simulink library "libbestfx"  (R2018b)
settings: Solver=VariableStepAuto  StartTime=0.0  StopTime=10.0  RelTol=1e-3
undefined symbols (not defined in the file or in its folder): R, S, VariantTypeR, VariantTypeS
libraries: simulink x25, $bdroot x14
(part 1 of 2)
settings Model: Creator=Timo Fix  LastModifiedBy=tfix

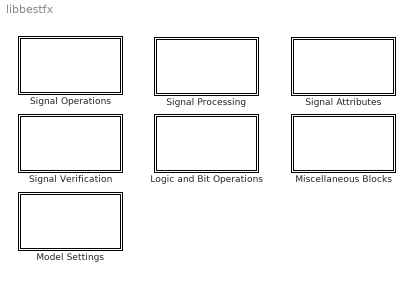
== system libbestfx ==
  Logic and Bit Operations : Subsystem
      mask Display:
      | color('white');
      | text(.1,.5,...
      |     ['\fontsize{18}me.'...
      |      '\fontsize{12}\fontname{courier}' newline ...
      |      'BitOps'],...
      |      'horizontalAlignment','left','texmode','on');
  Miscellaneous Blocks : Subsystem
      mask Display:
      | color('white');
      | text(.1,.5,...
      |     ['\fontsize{18}me.'...
      |      '\fontsize{12}\fontname{courier}' newline ...
      |      'Misc'],...
      |      'horizontalAlignment','left','texmode','on');
  Model Settings : Subsystem
      mask Display:
      | color('white');
      | text(.1,.5,...
      |     ['\fontsize{18}me.'...
      |      '\fontsize{12}\fontname{courier}' newline ...
      |      'Settings'],...
      |      'horizontalAlignment','left','texmode','on');
  Signal Attributes : Subsystem
      mask Display:
      | color('white');
      | text(.1,.5,...
      |     ['\fontsize{18}me.'...
      |      '\fontsize{12}\fontname{courier}' newline ...
      |      'SigAttr'],...
      |      'horizontalAlignment','left','texmode','on');
  Signal Operations : Subsystem
      mask Display:
      | color('white');
      | text(.1,.5,...
      |     ['\fontsize{18}me.'...
      |      '\fontsize{12}\fontname{courier}' newline ...
      |      'SigOps'],...
      |      'horizontalAlignment','left','texmode','on');
  Signal Processing : Subsystem
      mask Display:
      | color('white');
      | text(.1,.5,...
      |     ['\fontsize{18}me.'...
      |      '\fontsize{12}\fontname{courier}' newline ...
      |      'SigProc'],...
      |      'horizontalAlignment','left','texmode','on');
  Signal Verification : Subsystem
      mask Display:
      | color('white');
      | text(.1,.5,...
      |     ['\fontsize{18}me.'...
      |      '\fontsize{12}\fontname{courier}' newline ...
      |      'V&V'],...
      |      'horizontalAlignment','left','texmode','on');

== system libbestfx/Logic and Bit Operations ==
  Byte Creator : Subsystem  mask(ByteCreator me.){}
      mask help: Creates a byte composed of 8 bits.
      mask DialogControl ContainerLabel Prompt: Bit data width labels
      mask DialogControl TextLabelGroup1 Prompt: <b>Bit</b>: 1 bit<br> <b>Nibble</b>: 4 bits<br> <b>Byte</b>: 8 bits
      mask DialogControl TextLabelGroup2 Prompt: <b>Word</b>: 16 bits<br> <b>Double-Word</b>: 32 bits<br> <b>Long-Word</b>: 64 bits
  Byte Join : Subsystem  mask(ByteJoin me.){}
      mask help: Join two bytes to a word.
  Double-Word Creator : Subsystem  mask(DoubleWordCreator me.){}
      mask help: Creates a double-word composed of 32 bits.
      mask DialogControl ContainerLabel Prompt: Bit data width labels
      mask DialogControl TextLabelGroup1 Prompt: <b>Bit</b>: 1 bit<br> <b>Nibble</b>: 4 bits<br> <b>Byte</b>: 8 bits
      mask DialogControl TextLabelGroup2 Prompt: <b>Word</b>: 16 bits<br> <b>Double-Word</b>: 32 bits<br> <b>Long-Word</b>: 64 bits
  Double-Word Join : Subsystem  mask(DoubleWordJoin me.){}
      mask help: Join two double-words to a long-word.
  Nibble Creator : Subsystem  mask(NibbleCreator me.){}
      mask help: Creates a nibble composed of 4 bits.
      mask DialogControl ContainerLabel Prompt: Bit data width labels
      mask DialogControl TextLabelGroup1 Prompt: <b>Bit</b>: 1 bit<br> <b>Nibble</b>: 4 bits<br> <b>Byte</b>: 8 bits
      mask DialogControl TextLabelGroup2 Prompt: <b>Word</b>: 16 bits<br> <b>Double-Word</b>: 32 bits<br> <b>Long-Word</b>: 64 bits
  Nibble Join : Subsystem  mask(NibbleJoin me.){}
      mask help: Join two nibbles to a byte.
  Word Creator : Subsystem  mask(WordCreator me.){}
      mask help: Creates a word composed of 16 bits.
      mask DialogControl ContainerLabel Prompt: Bit data width labels
      mask DialogControl TextLabelGroup1 Prompt: <b>Bit</b>: 1 bit<br> <b>Nibble</b>: 4 bits<br> <b>Byte</b>: 8 bits
      mask DialogControl TextLabelGroup2 Prompt: <b>Word</b>: 16 bits<br> <b>Double-Word</b>: 32 bits<br> <b>Long-Word</b>: 64 bits
  Word Join : Subsystem  mask(WordJoin me.){}
      mask help: Join two words to a double-word.

== system libbestfx/Miscellaneous Blocks ==
  Continuous To Discrete : Subsystem  mask(ContinuousToDiscrete me.){Quantity=2, OutportDataType=Inherit: Inherit via back propagation, OutputPortSampleTime=-1}
      mask prompts: Quantity "Quantity Conversions:"; OutportDataType "Datatype of newly added outputs:"; OutputPortSampleTime "Output port sample time:"
      mask help: Convert continuous signals to discrete
      mask init:
      | me.sl.mask.ContinuousDiscrete();
      settings: CopyFcn=try;set(gcbh,'LinkStatus','none');end
      mask Display: plot([0 1], [0 1]);
  Discrete To Continuous : Subsystem  mask(DiscreteToContinuous me.){Quantity=2, OutportDataType=double, OutputPortSampleTime=-1}
      mask prompts: Quantity "Quantity Conversions:"; OutportDataType "Datatype of newly added outputs:"; OutputPortSampleTime "Output port sample time:"
      mask help: Convert discrete signals to continuous
      mask init:
      | me.sl.mask.ContinuousDiscrete();
      settings: CopyFcn=try;set(gcbh,'LinkStatus','none');end
      mask Display: plot([0 1], [0 1]);

== system libbestfx/Model Settings ==
  Design Block : Subsystem  InitFcn=|  mask(DesignBlock me.){blockver=V1.0}
      | if me.sl.style.DEBUG
      |     fprintf('%s::DesignBlock: apply style\n',me.sl.cfg.meSimulinkLibraryName());
      | end
      | me.sl.style.apply();
      mask prompts: blockver "Design Guideline Version"
      settings: OpenFcn=|
      | if me.sl.style.DEBUG
      |     fprintf('tsflib::DesignBlock: apply style\n');
      | end
      | me.sl.style.apply();
      mask TypeOptions blockver: V1.0
      mask Display:
      | color('black');
      | text(.1,.5,...
      |     ['\fontsize{18}me.'...
      |      '\fontsize{12}\fontname{courier}' newline ...
      |      'Apply Style'],...
      |      'horizontalAlignment','left','texmode','on');

== system libbestfx/Signal Attributes ==
  Data Pack : Subsystem  mask(DataPack .me){BlockSubtypeVariant=Unsigned, Length=8, Scale=1, Offset=0, ScaleDataType=Inherit: Inherit from 'Constant value', OffsetDataType=Inherit: Inherit from 'Constant value', OutputDataType=Inherit: Inherit via back propagation}
      mask prompts: BlockSubtypeVariant "Bit Specifier:"; Length "Length (Quantity Of Bits):"; Scale "Scale (Resolution Per Bit):"; Offset "Offset (Scaled):"; ScaleDataType "Scale:"; OffsetDataType "Offset:"
      mask help: Packs a physical or numerical signal (u) into a compressed equivalent in raw format (y, quantized signal with scaling and offset), using the specified parameters.
      mask init:
      | me.sl.mask.datapack();
      settings: AttributesFormatString=8 Unsigned Bits
      mask TypeOptions BlockSubtypeVariant: Unsigned | Signed | Floating-Point
      mask DialogControl TabParam Prompt: Main
      mask DialogControl Length Tooltip: Expect positive regular numeric value.
      mask DialogControl Scale Tooltip: Expect positive regular numeric value.
      mask DialogControl Offset Tooltip: Expect non-negative regular numeric value.
      mask DialogControl TabType Prompt: Parameter Attributes
      mask DialogControl TextType Prompt: The 'OutputDataType' specifies the desired datatype for this block. Please make sure that the data types of all parameters are identical.
      mask DialogControl TextTypeNote Prompt: <i style="color:blue">Note: In the case of back propagation, it should be considered that the numerical value in the runtime data type may not be represented correctly.</i>
      mask DialogControl TabMode Prompt: Info
      mask DialogControl TextModeCounter Prompt: <b>Counter:</b> Counts up immediately as soon as the counting unit has been activated, e.g. an 'Upper Limit' of ten is reached after nine counting steps.
      mask DialogControl TextModeTimer Prompt: <b>Timer:</b> Counts the elapsed counting steps when the counting unit is activated, e.g. an 'Upper Limit' of ten is reached after ten counting steps.
      mask DialogControl TextModeOptionFreeRunning Prompt: The option <b>Free-Running</b>: The counting unit is automatically reset after the status of the counting unit is active. The status is kept active for one cycle followed by a reset cycle.
      mask DialogControl TextModeOptionBidirectional Prompt: The option <b>Bidirectional</b>: After the status of the counting unit is active, it is held. The state is not reset to false until the count of the counting unit has dropped to zero again.
      mask DialogControl TextModeNote Prompt: <br><i style="color:blue;">Note: The internal counter and initial value cannot become negative, because they are saturated to zero.</i>
      mask Display: disp('pack');
  Data Unpack : Subsystem  mask(DataUnpack .me){BlockSubtypeVariant=Unsigned, Length=8, Scale=1, Offset=0, ScaleDataType=Inherit: Inherit from 'Constant value', OffsetDataType=Inherit: Inherit from 'Constant value', OutputDataType=Inherit: Inherit via back propagation}
      mask prompts: BlockSubtypeVariant "Bit Specifier:"; Length "Length (Quantity Of Bits):"; Scale "Scale (Resolution Per Bit):"; Offset "Offset (Scaled):"; ScaleDataType "Scale:"; OffsetDataType "Offset:"
      mask help: unpack a signal in raw format (u, quantized signal with scaling and offset) to its physical or numerical original equivalent (y), using the specified parameters.
      mask init:
      | me.sl.mask.datapack();
      settings: AttributesFormatString=8 Unsigned Bits
      mask TypeOptions BlockSubtypeVariant: Unsigned | Signed | Floating-Point
      mask DialogControl TabParam Prompt: Main
      mask DialogControl Length Tooltip: Expect positive regular numeric value.
      mask DialogControl Scale Tooltip: Expect positive regular numeric value.
      mask DialogControl Offset Tooltip: Expect non-negative regular numeric value.
      mask DialogControl TabType Prompt: Parameter Attributes
      mask DialogControl TextType Prompt: The 'Scale' specifies the desired datatype for this block. Please make sure that the data types of all parameters are identical.
      mask DialogControl TextTypeNote Prompt: <i style="color:blue">Note: In the case of back propagation, it should be considered that the numerical value in the runtime data type may not be represented correctly.</i>
      mask DialogControl TabMode Prompt: Info
      mask DialogControl TextModeCounter Prompt: <b>Counter:</b> Counts up immediately as soon as the counting unit has been activated, e.g. an 'Upper Limit' of ten is reached after nine counting steps.
      mask DialogControl TextModeTimer Prompt: <b>Timer:</b> Counts the elapsed counting steps when the counting unit is activated, e.g. an 'Upper Limit' of ten is reached after ten counting steps.
      mask DialogControl TextModeOptionFreeRunning Prompt: The option <b>Free-Running</b>: The counting unit is automatically reset after the status of the counting unit is active. The status is kept active for one cycle followed by a reset cycle.
      mask DialogControl TextModeOptionBidirectional Prompt: The option <b>Bidirectional</b>: After the status of the counting unit is active, it is held. The state is not reset to false until the count of the counting unit has dropped to zero again.
      mask DialogControl TextModeNote Prompt: <br><i style="color:blue;">Note: The internal counter and initial value cannot become negative, because they are saturated to zero.</i>
      mask Display: disp('unpack');
  Overwrite : Subsystem  mask(Overwrite .me){val=0.0}
      mask prompts: val "Overwrite value:"
      mask help: Overwrite the incoming signal value. Other signal properties like data type and dimension remain unchanged.
      mask Display: fprintf('y = %g',val)
  Rename : Subsystem  mask(Rename .me){}
      mask help: Renaming of the incoming signal. Other signal properties such as data type and dimension remain unchanged.
      mask Display: disp('rename');

== system libbestfx/Signal Operations ==
  Counter Timer Unit : Subsystem  mask(CounterTimerUnit .me){BlockSubtypeVariant=Counter, UpperLimitSourcePort=off, EnableSourcePort=on, IncrementSourcePort=off, DecrementSourcePort=off, InitialConditionSourcePort=off, ResetSourcePort=off, CounterTimerStateSinkPort=on, CounterTimerValueSinkPort=off, UpperLimit=10, Increment=1, Decrement=0, InitialCondition=0, UpperLimitDataType=Inherit: Inherit from 'Constant value', IncrementDataType=Inherit: Inherit from 'Constant value', DecrementDataType=Inherit: Inherit from 'Constant value', InitialConditionDataType=Inherit: Inherit from 'Constant value'}
      mask prompts: BlockSubtypeVariant "Mode:"; UpperLimitSourcePort "Show port 'Upper Limit'"; EnableSourcePort "Show port 'Enable'"; IncrementSourcePort "Show port 'Increment'"; DecrementSourcePort "Show port 'Decrement'"; InitialConditionSourcePort "Show port 'Initial Condition'"; ResetSourcePort "Show port 'Reset'"; CounterTimerStateSinkPort "Show port 'State'"; CounterTimerValueSinkPort "Show port 'Value'"; UpperLimit "Upper Limit:"; Increment "Counter Increment:"; Decrement "Counter Decrement:"; InitialCondition "Initial Condition: Limited to the value range from zero to the 'Upper Limit'."; UpperLimitDataType "Upper Limit:"; IncrementDataType "Increment:"; DecrementDataType "Decrement:"; InitialConditionDataType "Initial Condition:"
      mask help: Counter unit which counts in different ways. Two counting modes are available (counter/timer), each optionally with the option bidirectional or free-running.
      mask init:
      | me.sl.mask.countertimerunit();
      settings: AttributesFormatString=|
      | %<BlockSubtypeVariant>
      | Upper Limit: 10
      mask TypeOptions BlockSubtypeVariant: Counter | Timer | Bidirectional Counter | Bidirectional Timer | Free-Running Counter | Free-Running Timer
      mask DialogControl TabParam Prompt: Main
      mask DialogControl ContainerSources Prompt: Show Inports
      mask DialogControl ContainerSinks Prompt: Show Outports
      mask DialogControl UpperLimit Tooltip: Expect positive regular numeric value.
      mask DialogControl Increment Tooltip: Expect positive regular numeric value.
      mask DialogControl Decrement Tooltip: Expect non-negative regular numeric value.
      mask DialogControl InitialCondition Tooltip: Expect regular numeric value.
      mask DialogControl TabType Prompt: Parameter Attributes
      mask DialogControl TextType Prompt: The 'Upper Limit' specifies the desired datatype for the counting unit. Please make sure that the data types of all parameters are identical.
      mask DialogControl TextTypeNote Prompt: <i style="color:blue">Note: In the case of back propagation, it should be considered that the numerical value in the runtime data type may not be represented correctly.</i>
      mask DialogControl TabMode Prompt: Info
      mask DialogControl TextModeCounter Prompt: <b>Counter:</b> Counts up immediately as soon as the counting unit has been activated, e.g. an 'Upper Limit' of ten is reached after nine counting steps.
      mask DialogControl TextModeTimer Prompt: <b>Timer:</b> Counts the elapsed counting steps when the counting unit is activated, e.g. an 'Upper Limit' of ten is reached after ten counting steps.
      mask DialogControl TextModeOptionFreeRunning Prompt: The option <b>Free-Running</b>: The counting unit is automatically reset after the status of the counting unit is active. The status is kept active for one cycle followed by a reset cycle.
      mask DialogControl TextModeOptionBidirectional Prompt: The option <b>Bidirectional</b>: After the status of the counting unit is active, it is held. The state is not reset to false until the count of the counting unit has dropped to zero again.
      mask DialogControl TextModeNote Prompt: <br><i style="color:blue;">Note: The internal counter and initial value cannot become negative, because they are saturated to zero.</i>
  Debounce Unit : Subsystem  mask(CounterTimerUnit .me){BlockSubtypeVariant=Holding Element, SamplesSourcePort=off, Samples=10, SampleTime=-1, SamplesConversion=on, SamplesDataType=Inherit: Inherit from 'Constant value'}
      mask prompts: BlockSubtypeVariant "Mode:"; SamplesSourcePort "Show port 'Debounce Samples'"; Samples "Debounce Samples:"; SampleTime "Sample Time:"; SamplesConversion "Convert 'Debounce Samples' to time interval in seconds"; SamplesDataType "Debounce Samples:"
      mask help: Debouncing unit that suppresses fast changes of the input signal (u) in various ways. Three modes are available (holding element, switch-on delay and switch-off delay).
      mask init:
      | me.sl.mask.debounceunit();
      settings: AttributesFormatString=|
      | %<BlockSubtypeVariant>
      | 10x samples
      mask TypeOptions BlockSubtypeVariant: Holding Element | Switch-On Delay | Switch-Off Delay
      mask DialogControl TabParam Prompt: Main
      mask DialogControl ContainerSources Prompt: Show Inports
      mask DialogControl Samples Tooltip: Expect positive regular numeric value.
      mask DialogControl ContainerPreview Prompt: Block Parameter Preview
      mask DialogControl TextPreviewNote Prompt: <i style="color:blue">Note: A conversion is only possible if the 'Sample Time' is explicitly specified, which means it is not '-1'.</i>
      mask DialogControl TabType Prompt: Parameter Attributes
      mask DialogControl TabMode Prompt: Info
      mask DialogControl TextModeHoldingElement Prompt: <b>Holding Element:</b> Holds the active level for a presettable 'Debounce Samples' minimum time. After this minimum time has elapsed, the input level is passed through.
      mask DialogControl TextModeSwitchOffDelay Prompt: <b>Switch-Off Delay:</b> Holds the active level for a presettable 'Debounce Samples' hold time after the input signal is reset. The duration of this hold time restarts with each falling edge.
      mask DialogControl TextModeSwitchOnDelay Prompt: <b>Switch-On Delay:</b> Suppresses the active level of the input signal until the predefinable 'Debounce Samples' hold time has elapsed.
  Flip-Flop : Subsystem  mask(FlipFlop .me){BlockSubtypeVariant=Bistable S-R, StateSourcePort=on, NegatedStateSourcePort=off, InitialCondition=false}
      mask prompts: BlockSubtypeVariant "Mode:"; StateSourcePort "Show port 'State'"; NegatedStateSourcePort "Show port 'Negated State'"; InitialCondition "Initial Condition:"
      mask help: Bistable flip-flop without restricted combination (forbidden state). Set or reset condition is dominant as soon as both inputs are set. Two flip-flop modes are available.
      mask init:
      | me.sl.mask.flipflop();
      settings: AttributesFormatString=%<BlockSubtypeVariant>
      mask TypeOptions BlockSubtypeVariant: Bistable S-R | Bistable R-S
      mask DialogControl TabParam Prompt: Main
      mask DialogControl ContainerSinks Prompt: Show Outports
      mask DialogControl TabMode Prompt: Info
      mask DialogControl TextModeSR Prompt: <b>Bistable S-R:</b> Characterized by a dominant set condition.
      mask DialogControl TextModeRS Prompt: <b>Bistable R-S:</b> Characterized by a dominant reset condition.
      mask Display:
      | color('green');
      | port_label('input', 1, '_');
  Interactive Switch : Subsystem  mask(InteractiveSwitch .me){ctrl=off}
      mask prompts: ctrl "BUTTON"
      mask init:
      | me.sl.mask.switchinteractive();
      settings: OpenFcn=me.sl.mask.switchinteractive('clbk','openfnc')
      mask Display: disp('OFF')
  Pulse Divider : Subsystem  mask(PulseDivider me.){DivisorSourcePort=off, Divisor=2, DivisorDataType=uint8}
      mask prompts: DivisorSourcePort "Show port "Divisor""; DivisorDataType "Divisor:"
      mask help: The sequence of input pulses (u) is reduced by the divisor (k), resulting in slower output pulses (y).
      mask init:
      | me.sl.mask.pulsedivider();
      mask DialogControl TabParam Prompt: Main
      mask DialogControl ContainerSource Prompt: Show Inports
      mask DialogControl TabTypes Prompt: Parameter Attributes
  Pulse Selector : Subsystem  mask(PulseSelector me.){MaximumSourcePort=off, SubsetSourcePort=off, Maximum=5, Subset=3, MaximumDataType=uint8, SubsetDataType=uint8}
      mask prompts: MaximumSourcePort "Show port "Maximum Of Pulses""; SubsetSourcePort "Show port "Subset Of Pulses""; Maximum "Total Amount:"; Subset "Subset Amount: Limited to the value range from zero to the 'Total Amount'"; MaximumDataType "Maximum Of Pulses:"; SubsetDataType "Subset Of Pulses:"
      mask help: Starting from an ever-repeating sequence of input pulses (u), the length of the sequence is described by the maximum of pulses (nmax). Only a subset of pulses (n) are passed through. Intervening pulses are suppressed until the sequence starts from the beginning.
      mask init:
      | me.sl.mask.pulseselector();
      settings: AttributesFormatString=3 out of 5
      mask DialogControl TabParam Prompt: Main
      mask DialogControl ContainerSource Prompt: Show Inports
      mask DialogControl TabTypes Prompt: Parameter Attributes
  Switch To Zero : Subsystem  mask(SwitchToZero me.){}
      mask help: Sets the output signal (y) to zero if the input signal (TF) is set. Otherwise the input signal (u) is passed through.
      mask Display: fprintf('Zero when\nTF > 0');

== system libbestfx/Signal Processing ==
  Discrete Filter : Subsystem  mask(DiscreteFilter .me){BlockSubtypeVariant=Lowpass, FilterCoefficientSourcePort=off, InitialConditionSourcePort=off, ResetSourcePort=off, FilterCoefficient=0.97, InitialCondition=0, FilterCoefficientDataType=Inherit: Inherit from 'Constant value', InitialConditionDataType=Inherit: Inherit from 'Constant value'}
      mask prompts: BlockSubtypeVariant "Mode:"; FilterCoefficientSourcePort "Show port 'Filter Coefficient'"; InitialConditionSourcePort "Show port 'Initial Condition'"; ResetSourcePort "Show port 'Reset'"; FilterCoefficient "Filter Coefficent [0..1]:"; InitialCondition "Initial Condition:"; FilterCoefficientDataType "Filter Coefficent:"; InitialConditionDataType "Initial Condition:"
      mask help: Digital discrete signal filter. Two modes are available (lowpass/highpass).
      mask init:
      | me.sl.mask.discretefilter();
      settings: AttributesFormatString=|
      | %<BlockSubtypeVariant>
      | Filter Coefficient: 0.97
      mask TypeOptions BlockSubtypeVariant: Lowpass | Highpass
      mask DialogControl TabParam Prompt: Main
      mask DialogControl ContainerShowPorts Prompt: Show Inports
      mask DialogControl TabType Prompt: Parameter Attributes
      mask DialogControl TabMode Prompt: Info
      mask DialogControl ContainerMode Prompt: Filter Transfer Functions
      mask DialogControl TextModeLowpass Prompt: Discrete Lowpass:
      mask DialogControl TextModeHighpass Prompt: Discrete Highpass:
      mask DialogControl TextModeLowpassTransferFunction Prompt: <table><td><code><br>LP(z)=<br></code></td><td><code>1-T<br>----<br>z -T</code></td></table>
      mask DialogControl TextModeHighpassTransferFunction Prompt: <table><td><code><br>HP(z)=<br></code></td><td><code>z -1<br>----<br>z -T</code></td></table>
      mask Display: disp('LP(z)');

== system libbestfx/Signal Verification ==
  Validate : Subsystem  mask{BlockSubtypeVariant=Value Inside, LowerLimitSourcePort=off, UpperLimitSourcePort=off, LowerLimit=0, UpperLimit=1, LowerLimitDataType=Inherit: Inherit from 'Constant value', UpperLimitDataType=Inherit: Inherit from 'Constant value'}
      mask prompts: BlockSubtypeVariant "Mode:"; LowerLimitSourcePort "Show port 'Lower Limit'"; UpperLimitSourcePort "Show port 'Upper Limit'"; LowerLimit "Lower Limit:"; UpperLimit "Upper Limit:"; LowerLimitDataType "Lower Limit:"; UpperLimitDataType "Upper Limit:"
      mask init:
      | me.sl.mask.validate();
      settings: AttributesFormatString=|
      | %<BlockSubtypeVariant>
      | Interval [0 .. 1]
      mask TypeOptions BlockSubtypeVariant: Value Inside | Value Below | Value Above | Stuck | Stuck Inside | Stuck Below | Stuck Above
      mask DialogControl TabParam Prompt: Main
      mask DialogControl ContainerSources Prompt: Show Inports
      mask DialogControl ContainerSinks Prompt: Show Outports
      mask DialogControl TabType Prompt: Parameter Attributes

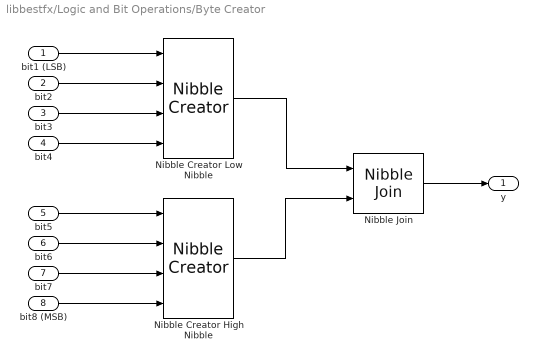
== system libbestfx/Logic and Bit Operations/Byte Creator ==
  bit1 (LSB) : Inport
  bit2 : Inport  Port=2
  bit3 : Inport  Port=3
  bit4 : Inport  Port=4
  bit5 : Inport  Port=5
  bit6 : Inport  Port=6
  bit7 : Inport  Port=7
  bit8 (MSB) : Inport  Port=8
  Nibble Creator High Nibble : $bdroot/Logic and Bit Operations/Nibble Creator
  Nibble Creator Low Nibble : $bdroot/Logic and Bit Operations/Nibble Creator
  Nibble Join : $bdroot/Logic and Bit Operations/Nibble Join
  y : Outport
  wires:
  Nibble Creator High Nibble/1 -> Nibble Join/2
  Nibble Creator Low Nibble/1 -> Nibble Join/1
  bit8 (MSB)/1 -> Nibble Creator High Nibble/4
  bit7/1 -> Nibble Creator High Nibble/3
  bit6/1 -> Nibble Creator High Nibble/2
  bit5/1 -> Nibble Creator High Nibble/1
  bit4/1 -> Nibble Creator Low Nibble/4
  bit3/1 -> Nibble Creator Low Nibble/3
  Nibble Join/1 -> y/1
  bit2/1 -> Nibble Creator Low Nibble/2
  bit1 (LSB)/1 -> Nibble Creator Low Nibble/1

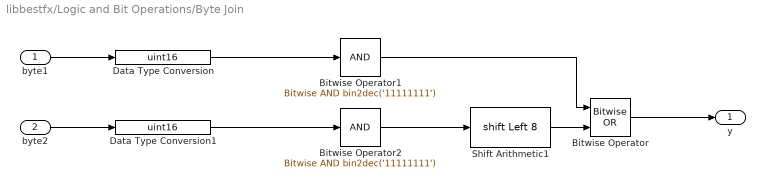
== system libbestfx/Logic and Bit Operations/Byte Join ==
  "byte1 " : Inport
  byte2 : Inport  Port=2
  Bitwise Operator : simulink/Logic and Bit Operations/Bitwise Operator  logicop=OR  UseBitMask=off  NumInputPorts=2  BitMask=bin2dec('11011001')  BitMaskRealWorld=Stored Integer
  Bitwise Operator1 : simulink/Logic and Bit Operations/Bitwise Operator  logicop=AND  UseBitMask=on  BitMask=bin2dec('11111111')  BitMaskRealWorld=Stored Integer
  Bitwise Operator2 : simulink/Logic and Bit Operations/Bitwise Operator  logicop=AND  UseBitMask=on  BitMask=bin2dec('11111111')  BitMaskRealWorld=Stored Integer
  Data Type Conversion : DataTypeConversion  OutDataTypeStr=uint16
  Data Type Conversion1 : DataTypeConversion  OutDataTypeStr=uint16
  Shift Arithmetic1 : ArithShift  BitShiftNumber=8  BitShiftDirection=Left
  y : Outport
  wires:
  byte2/1 -> Data Type Conversion1/1
  Bitwise Operator2/1 -> Shift Arithmetic1/1
  Shift Arithmetic1/1 -> Bitwise Operator/2
  Bitwise Operator1/1 -> Bitwise Operator/1
  Bitwise Operator/1 -> y/1
  Data Type Conversion/1 -> Bitwise Operator1/1
  "byte1 "/1 -> Data Type Conversion/1
  Data Type Conversion1/1 -> Bitwise Operator2/1

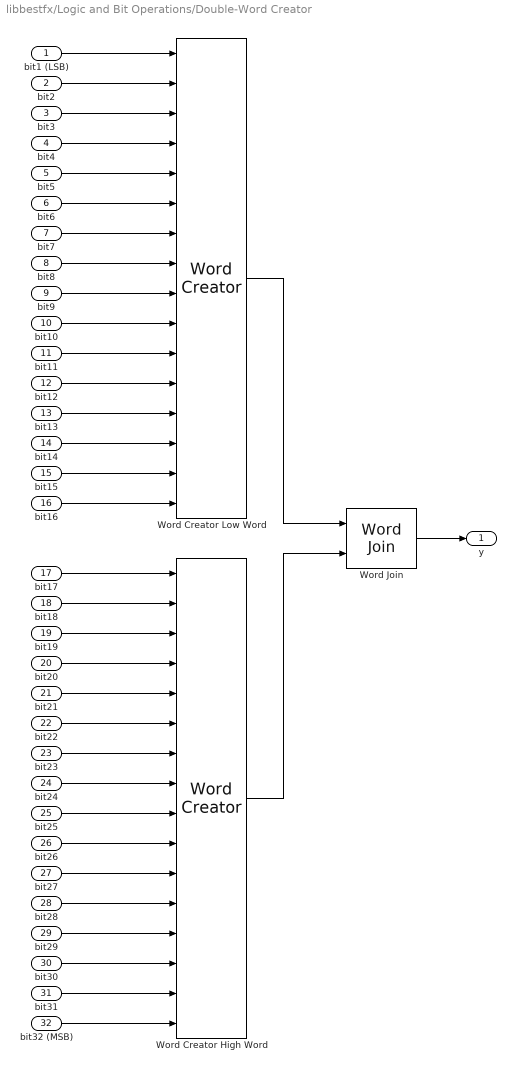
== system libbestfx/Logic and Bit Operations/Double-Word Creator ==
  bit1 (LSB) : Inport
  bit2 : Inport  Port=2
  bit3 : Inport  Port=3
  bit4 : Inport  Port=4
  bit5 : Inport  Port=5
  bit6 : Inport  Port=6
  bit7 : Inport  Port=7
  bit8 : Inport  Port=8
  bit9 : Inport  Port=9
  bit10 : Inport  Port=10
  bit11 : Inport  Port=11
  bit12 : Inport  Port=12
  bit13 : Inport  Port=13
  bit14 : Inport  Port=14
  bit15 : Inport  Port=15
  bit16 : Inport  Port=16
  bit17 : Inport  Port=17
  bit18 : Inport  Port=18
  bit19 : Inport  Port=19
  bit20 : Inport  Port=20
  bit21 : Inport  Port=21
  bit22 : Inport  Port=22
  bit23 : Inport  Port=23
  bit24 : Inport  Port=24
  bit25 : Inport  Port=25
  bit26 : Inport  Port=26
  bit27 : Inport  Port=27
  bit28 : Inport  Port=28
  bit29 : Inport  Port=29
  bit30 : Inport  Port=30
  bit31 : Inport  Port=31
  bit32 (MSB) : Inport  Port=32
  Word Creator High Word : $bdroot/Logic and Bit Operations/Word Creator
  Word Creator Low Word : $bdroot/Logic and Bit Operations/Word Creator
  Word Join : $bdroot/Logic and Bit Operations/Word Join
  y : Outport
  wires:
  bit1 (LSB)/1 -> Word Creator Low Word/1
  Word Creator High Word/1 -> Word Join/2
  Word Creator Low Word/1 -> Word Join/1
  Word Join/1 -> y/1
  bit2/1 -> Word Creator Low Word/2
  bit3/1 -> Word Creator Low Word/3
  bit4/1 -> Word Creator Low Word/4
  bit5/1 -> Word Creator Low Word/5
  bit6/1 -> Word Creator Low Word/6
  bit7/1 -> Word Creator Low Word/7
  bit8/1 -> Word Creator Low Word/8
  bit9/1 -> Word Creator Low Word/9
  bit10/1 -> Word Creator Low Word/10
  bit11/1 -> Word Creator Low Word/11
  bit12/1 -> Word Creator Low Word/12
  bit13/1 -> Word Creator Low Word/13
  bit14/1 -> Word Creator Low Word/14
  bit15/1 -> Word Creator Low Word/15
  bit16/1 -> Word Creator Low Word/16
  bit17/1 -> Word Creator High Word/1
  bit18/1 -> Word Creator High Word/2
  bit19/1 -> Word Creator High Word/3
  bit20/1 -> Word Creator High Word/4
  bit21/1 -> Word Creator High Word/5
  bit22/1 -> Word Creator High Word/6
  bit23/1 -> Word Creator High Word/7
  bit24/1 -> Word Creator High Word/8
  bit25/1 -> Word Creator High Word/9
  bit26/1 -> Word Creator High Word/10
  bit27/1 -> Word Creator High Word/11
  bit28/1 -> Word Creator High Word/12
  bit29/1 -> Word Creator High Word/13
  bit30/1 -> Word Creator High Word/14
  bit31/1 -> Word Creator High Word/15
  bit32 (MSB)/1 -> Word Creator High Word/16

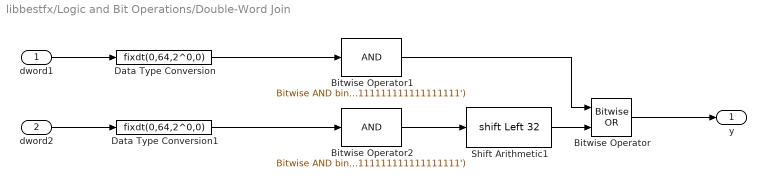
== system libbestfx/Logic and Bit Operations/Double-Word Join ==
  "dword1 " : Inport
  dword2 : Inport  Port=2
  Bitwise Operator : simulink/Logic and Bit Operations/Bitwise Operator  logicop=OR  UseBitMask=off  NumInputPorts=2  BitMask=bin2dec('11011001')  BitMaskRealWorld=Stored Integer
  Bitwise Operator1 : simulink/Logic and Bit Operations/Bitwise Operator  logicop=AND  UseBitMask=on  BitMask=bin2dec('11111111111111111111111111111111')  BitMaskRealWorld=Stored Integer
  Bitwise Operator2 : simulink/Logic and Bit Operations/Bitwise Operator  logicop=AND  UseBitMask=on  BitMask=bin2dec('11111111111111111111111111111111')  BitMaskRealWorld=Stored Integer
  Data Type Conversion : DataTypeConversion  OutDataTypeStr=fixdt(0,64,2^0,0)
  Data Type Conversion1 : DataTypeConversion  OutDataTypeStr=fixdt(0,64,2^0,0)
  Shift Arithmetic1 : ArithShift  BitShiftNumber=32  BitShiftDirection=Left
  y : Outport
  wires:
  Data Type Conversion1/1 -> Bitwise Operator2/1
  "dword1 "/1 -> Data Type Conversion/1
  Data Type Conversion/1 -> Bitwise Operator1/1
  Bitwise Operator/1 -> y/1
  Bitwise Operator1/1 -> Bitwise Operator/1
  Shift Arithmetic1/1 -> Bitwise Operator/2
  Bitwise Operator2/1 -> Shift Arithmetic1/1
  dword2/1 -> Data Type Conversion1/1

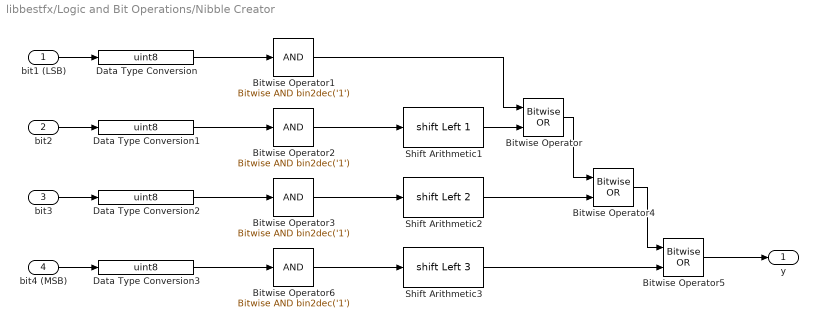
== system libbestfx/Logic and Bit Operations/Nibble Creator ==
  bit1 (LSB) : Inport
  bit2 : Inport  Port=2
  bit3 : Inport  Port=3
  bit4 (MSB) : Inport  Port=4
  Bitwise Operator : simulink/Logic and Bit Operations/Bitwise Operator  logicop=OR  UseBitMask=off  NumInputPorts=2  BitMask=bin2dec('11011001')  BitMaskRealWorld=Stored Integer
  Bitwise Operator{1..3,6} (4 alike) : simulink/Logic and Bit Operations/Bitwise Operator  logicop=AND  UseBitMask=on  BitMask=bin2dec('1')  BitMaskRealWorld=Stored Integer
  Bitwise Operator4 : simulink/Logic and Bit Operations/Bitwise Operator  logicop=OR  UseBitMask=off  NumInputPorts=2  BitMask=bin2dec('11011001')  BitMaskRealWorld=Stored Integer
  Bitwise Operator5 : simulink/Logic and Bit Operations/Bitwise Operator  logicop=OR  UseBitMask=off  NumInputPorts=2  BitMask=bin2dec('11011001')  BitMaskRealWorld=Stored Integer
  Data Type Conversion{,1..3} (4 alike) : DataTypeConversion  OutDataTypeStr=uint8
  Shift Arithmetic1 : ArithShift  BitShiftNumber=1  BitShiftDirection=Left
  Shift Arithmetic2 : ArithShift  BitShiftNumber=2  BitShiftDirection=Left
  Shift Arithmetic3 : ArithShift  BitShiftNumber=3  BitShiftDirection=Left
  y : Outport
  wires:
  bit1 (LSB)/1 -> Data Type Conversion/1
  bit2/1 -> Data Type Conversion1/1
  Bitwise Operator2/1 -> Shift Arithmetic1/1
  Bitwise Operator/1 -> Bitwise Operator4/1
  Shift Arithmetic1/1 -> Bitwise Operator/2
  Bitwise Operator1/1 -> Bitwise Operator/1
  Bitwise Operator3/1 -> Shift Arithmetic2/1
  bit3/1 -> Data Type Conversion2/1
  Shift Arithmetic2/1 -> Bitwise Operator4/2
  Shift Arithmetic3/1 -> Bitwise Operator5/2
  bit4 (MSB)/1 -> Data Type Conversion3/1
  Bitwise Operator6/1 -> Shift Arithmetic3/1
  Bitwise Operator4/1 -> Bitwise Operator5/1
  Bitwise Operator5/1 -> y/1
  Data Type Conversion/1 -> Bitwise Operator1/1
  Data Type Conversion1/1 -> Bitwise Operator2/1
  Data Type Conversion2/1 -> Bitwise Operator3/1
  Data Type Conversion3/1 -> Bitwise Operator6/1

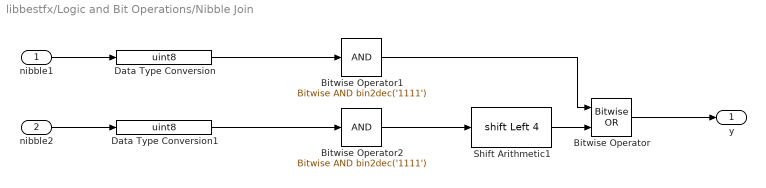
== system libbestfx/Logic and Bit Operations/Nibble Join ==
  "nibble1 " : Inport
  nibble2 : Inport  Port=2
  Bitwise Operator : simulink/Logic and Bit Operations/Bitwise Operator  logicop=OR  UseBitMask=off  NumInputPorts=2  BitMask=bin2dec('11011001')  BitMaskRealWorld=Stored Integer
  Bitwise Operator1 : simulink/Logic and Bit Operations/Bitwise Operator  logicop=AND  UseBitMask=on  BitMask=bin2dec('1111')  BitMaskRealWorld=Stored Integer
  Bitwise Operator2 : simulink/Logic and Bit Operations/Bitwise Operator  logicop=AND  UseBitMask=on  BitMask=bin2dec('1111')  BitMaskRealWorld=Stored Integer
  Data Type Conversion : DataTypeConversion  OutDataTypeStr=uint8
  Data Type Conversion1 : DataTypeConversion  OutDataTypeStr=uint8
  Shift Arithmetic1 : ArithShift  BitShiftNumber=4  BitShiftDirection=Left
  y : Outport
  wires:
  nibble2/1 -> Data Type Conversion1/1
  Bitwise Operator2/1 -> Shift Arithmetic1/1
  Shift Arithmetic1/1 -> Bitwise Operator/2
  Bitwise Operator1/1 -> Bitwise Operator/1
  Bitwise Operator/1 -> y/1
  Data Type Conversion/1 -> Bitwise Operator1/1
  "nibble1 "/1 -> Data Type Conversion/1
  Data Type Conversion1/1 -> Bitwise Operator2/1

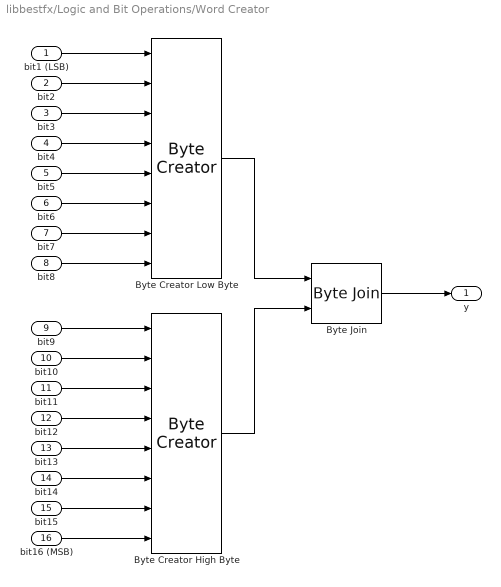
== system libbestfx/Logic and Bit Operations/Word Creator ==
  bit1 (LSB) : Inport
  bit2 : Inport  Port=2
  bit3 : Inport  Port=3
  bit4 : Inport  Port=4
  bit5 : Inport  Port=5
  bit6 : Inport  Port=6
  bit7 : Inport  Port=7
  bit8 : Inport  Port=8
  bit9 : Inport  Port=9
  bit10 : Inport  Port=10
  bit11 : Inport  Port=11
  bit12 : Inport  Port=12
  bit13 : Inport  Port=13
  bit14 : Inport  Port=14
  bit15 : Inport  Port=15
  bit16 (MSB) : Inport  Port=16
  Byte Creator High Byte : $bdroot/Logic and Bit Operations/Byte Creator
  Byte Creator Low Byte : $bdroot/Logic and Bit Operations/Byte Creator
  Byte Join : $bdroot/Logic and Bit Operations/Byte Join
  y : Outport
  wires:
  Byte Creator Low Byte/1 -> Byte Join/1
  Byte Creator High Byte/1 -> Byte Join/2
  bit1 (LSB)/1 -> Byte Creator Low Byte/1
  Byte Join/1 -> y/1
  bit2/1 -> Byte Creator Low Byte/2
  bit3/1 -> Byte Creator Low Byte/3
  bit4/1 -> Byte Creator Low Byte/4
  bit5/1 -> Byte Creator Low Byte/5
  bit6/1 -> Byte Creator Low Byte/6
  bit7/1 -> Byte Creator Low Byte/7
  bit8/1 -> Byte Creator Low Byte/8
  bit9/1 -> Byte Creator High Byte/1
  bit10/1 -> Byte Creator High Byte/2
  bit11/1 -> Byte Creator High Byte/3
  bit12/1 -> Byte Creator High Byte/4
  bit13/1 -> Byte Creator High Byte/5
  bit14/1 -> Byte Creator High Byte/6
  bit15/1 -> Byte Creator High Byte/7
  bit16 (MSB)/1 -> Byte Creator High Byte/8

== system libbestfx/Logic and Bit Operations/Word Join ==
  "word1 " : Inport
  word2 : Inport  Port=2
  Bitwise Operator : simulink/Logic and Bit Operations/Bitwise Operator  logicop=OR  UseBitMask=off  NumInputPorts=2  BitMask=bin2dec('11011001')  BitMaskRealWorld=Stored Integer
  Bitwise Operator1 : simulink/Logic and Bit Operations/Bitwise Operator  logicop=AND  UseBitMask=on  BitMask=bin2dec('1111111111111111')  BitMaskRealWorld=Stored Integer
  Bitwise Operator2 : simulink/Logic and Bit Operations/Bitwise Operator  logicop=AND  UseBitMask=on  BitMask=bin2dec('1111111111111111')  BitMaskRealWorld=Stored Integer
  Data Type Conversion : DataTypeConversion  OutDataTypeStr=uint32
  Data Type Conversion1 : DataTypeConversion  OutDataTypeStr=uint32
  Shift Arithmetic1 : ArithShift  BitShiftNumber=16  BitShiftDirection=Left
  y : Outport
  wires:
  Data Type Conversion1/1 -> Bitwise Operator2/1
  "word1 "/1 -> Data Type Conversion/1
  Data Type Conversion/1 -> Bitwise Operator1/1
  Bitwise Operator/1 -> y/1
  Bitwise Operator1/1 -> Bitwise Operator/1
  Shift Arithmetic1/1 -> Bitwise Operator/2
  Bitwise Operator2/1 -> Shift Arithmetic1/1
  word2/1 -> Data Type Conversion1/1

== system libbestfx/Miscellaneous Blocks/Continuous To Discrete ==
  u1 : Inport
  u2 : Inport  Port=2
  DataTypeConversion1 : DataTypeConversion  SaturateOnIntegerOverflow=on  RndMeth=Zero
  DataTypeConversion2 : DataTypeConversion  SaturateOnIntegerOverflow=on  RndMeth=Zero
  RateTransition1 : RateTransition  OutPortSampleTime=OutputPortSampleTime
  RateTransition2 : RateTransition  OutPortSampleTime=OutputPortSampleTime
  y1 : Outport
  y2 : Outport  Port=2
  wires:
  u1/1 -> RateTransition1/1
  RateTransition1/1 -> DataTypeConversion1/1
  DataTypeConversion1/1 -> y1/1
  u2/1 -> RateTransition2/1
  RateTransition2/1 -> DataTypeConversion2/1
  DataTypeConversion2/1 -> y2/1

== system libbestfx/Miscellaneous Blocks/Discrete To Continuous ==
  u1 : Inport
  u2 : Inport  Port=2
  DataTypeConversion1 : DataTypeConversion  OutDataTypeStr=double  SaturateOnIntegerOverflow=on  RndMeth=Zero
  DataTypeConversion2 : DataTypeConversion  OutDataTypeStr=double  SaturateOnIntegerOverflow=on  RndMeth=Zero
  RateTransition1 : RateTransition  OutPortSampleTime=OutputPortSampleTime
  RateTransition2 : RateTransition  OutPortSampleTime=OutputPortSampleTime
  y1 : Outport
  y2 : Outport  Port=2
  wires:
  u1/1 -> RateTransition1/1
  RateTransition1/1 -> DataTypeConversion1/1
  DataTypeConversion1/1 -> y1/1
  u2/1 -> RateTransition2/1
  RateTransition2/1 -> DataTypeConversion2/1
  DataTypeConversion2/1 -> y2/1

== system libbestfx/Model Settings/Design Block ==
  Empty : Subsystem

== system libbestfx/Signal Attributes/Data Pack ==
  u : Inport
  Offset : Constant  Value=Offset  OutDataTypeStr=OffsetDataType
  Product : Product  Inputs=*/  OutDataTypeStr=OutputDataType
  Quantizer : Quantizer  QuantizationInterval=Scale
  Scale : Constant  Value=Scale  OutDataTypeStr=ScaleDataType
  Sum : Sum  Inputs=|+-
  VariantSpecifier : Subsystem  VariantControlMode=Label  Variant=on  VariantControl=Variant1  LabelModeActiveChoice=VariantSpecifierUnsigned
  y : Outport
  wires:
  Offset/1 -> Sum/2
  Scale/1 -> Product/2
  Sum/1 -> Quantizer/1
  Product/1 -> VariantSpecifier/1("u ")
  VariantSpecifier/1(" y") -> y/1
  u/1 -> Sum/1
  Quantizer/1 -> Product/1

== system libbestfx/Signal Attributes/Data Unpack ==
  u : Inport
  Offset : Constant  Value=Offset  OutDataTypeStr=OffsetDataType
  Product : Product  OutDataTypeStr=OutputDataType
  Scale : Constant  Value=Scale  OutDataTypeStr=ScaleDataType
  Sum : Sum  Inputs=|++  OutDataTypeStr=OutputDataType
  VariantSpecifier : Subsystem  VariantControlMode=Label  Variant=on  VariantControl=Variant1  LabelModeActiveChoice=VariantSpecifierUnsigned
  y : Outport
  wires:
  Product/1 -> Sum/1
  Offset/1 -> Sum/2
  u/1 -> VariantSpecifier/1("u ")
  VariantSpecifier/1(" y") -> Product/1
  Scale/1 -> Product/2
  Sum/1 -> y/1

== system libbestfx/Signal Attributes/Overwrite ==
  u : Inport
  Constant : Constant  Value=val  OutDataTypeStr=Inherit: Inherit via back propagation
  Data Type Duplicate : DataTypeDuplicate
  Terminator : Terminator
  y : Outport
  wires:
  u/1 -> Data Type Duplicate/1, Terminator/1
  Constant/1 -> Data Type Duplicate/2, y/1

== system libbestfx/Signal Attributes/Rename ==
  u : Inport
  rename : Gain  OutDataTypeStr=Inherit: Same as input  ParamDataTypeStr=Inherit: Same as input
  y : Outport
  wires:
  rename/1 -> y/1
  u/1 -> rename/1

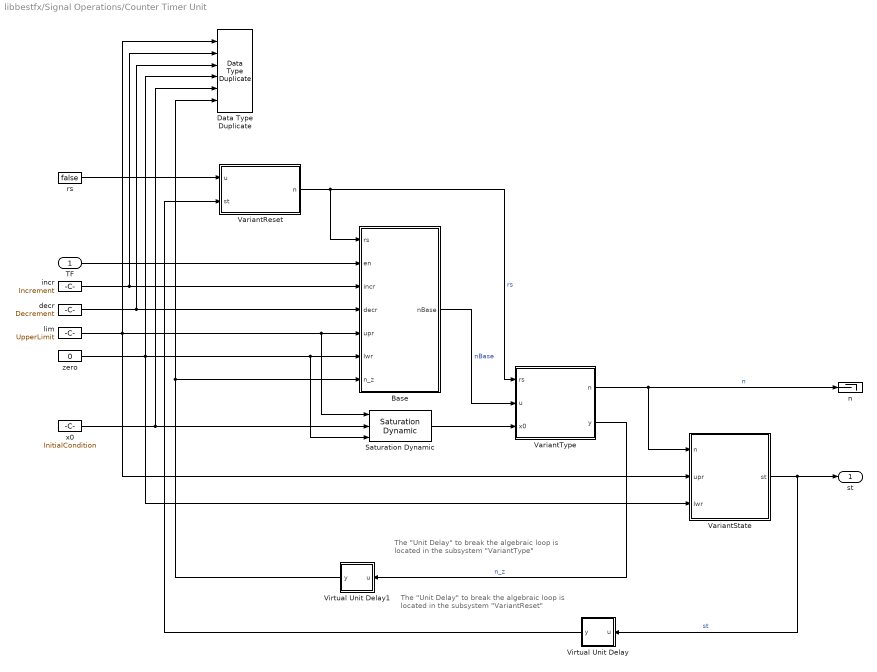
== system libbestfx/Signal Operations/Counter Timer Unit ==
  note: The "Unit Delay" to break the algebraic loop
      | is located in the subsystem "VariantType"
  note: The "Unit Delay" to break the algebraic loop
      | is located in the subsystem "VariantReset"
  TF : Inport
  Base : Subsystem
  Data Type Duplicate : DataTypeDuplicate  NumInputPorts=6
  Saturation Dynamic : simulink/Discontinuities/Saturation Dynamic  OutMin=[]  OutMax=[]  OutDataTypeStr=Inherit: Same as second input  OutDataType=fixdt(1, 16)  OutScaling=2^-10  DoSatur=off
  VariantReset : Subsystem  VariantControlMode=Label  Variant=on  LabelModeActiveChoice=VariantResetPassThrough
  VariantState : Subsystem  VariantControlMode=Label  Variant=on  LabelModeActiveChoice=VariantStateLevel
  VariantType : Subsystem  VariantControlMode=Label  Variant=on  LabelModeActiveChoice=VariantTypeCounter
  Virtual Unit Delay : Subsystem  mask(Virtual Unit Delay){}
      settings: AttributesFormatString=block has no effect
      mask Display: disp('1/z')
  Virtual Unit Delay1 : Subsystem  mask(Virtual Unit Delay){}
      settings: AttributesFormatString=block has no effect
      mask Display: disp('1/z')
  decr : Constant  Value=Decrement  OutDataTypeStr=DecrementDataType
  incr : Constant  Value=Increment  OutDataTypeStr=IncrementDataType
  lim : Constant  Value=UpperLimit  OutDataTypeStr=UpperLimitDataType
  n : Terminator
  rs : Constant  Value=false
  x0 : Constant  Value=InitialCondition  OutDataTypeStr=InitialConditionDataType
  zero : Constant  Value=0  OutDataTypeStr=Inherit: Inherit via back propagation
  st : Outport
  wires:
  Saturation Dynamic/1 -> VariantType/3(x0)
  TF/1 -> Base/2(en)
  Base/1(nBase) -> VariantType/2(u)  "nBase"
  lim/1 -> Data Type Duplicate/1, Base/5(upr), Saturation Dynamic/1, VariantState/2(upr)
  VariantState/1(st) -> Virtual Unit Delay/1(u), st/1  "st"
  zero/1 -> Data Type Duplicate/4, Base/6(lwr), Saturation Dynamic/3, VariantState/3(lwr)
  VariantType/1(n) -> n/1, VariantState/1(n)  "n"
  VariantType/2(y) -> Virtual Unit Delay1/1(u)  "n_z"
  incr/1 -> Data Type Duplicate/2, Base/3(incr)
  x0/1 -> Data Type Duplicate/5, Saturation Dynamic/2
  VariantReset/1(n) -> Base/1(rs), VariantType/1(rs)  "rs"
  decr/1 -> Data Type Duplicate/3, Base/4(decr)
  Virtual Unit Delay/1(y) -> VariantReset/2(st)
  Virtual Unit Delay1/1(y) -> Base/7(n_z), Data Type Duplicate/6
  rs/1 -> VariantReset/1(u)

== system libbestfx/Signal Operations/Debounce Unit ==
  note: The "Unit Delay" to break the algebraic loop
      | is located in the subsystem "Counter"
  u : Inport  SampleTime=SampleTime
  Count : Subsystem  VariantControl=Variant1
  Flip-Flop : $bdroot/Signal Operations/Flip-Flop  BlockSubtypeVariant=Bistable S-R  StateSourcePort=on  NegatedStateSourcePort=off  InitialCondition=false
      settings: AttributesFormatString=%<BlockSubtypeVariant>
  OR : Logic  Operator=OR  AllPortsSameDT=off  OutDataTypeStr=boolean
  VariantControl : Subsystem  VariantControlMode=Label  Variant=on  VariantControl=Variant1  LabelModeActiveChoice=VariantControlNoReset
  VariantDebounce : Subsystem  VariantControlMode=Label  Variant=on  VariantControl=Variant1  LabelModeActiveChoice=VariantDebounceCaptureHold
  Virtual Unit Delay : Subsystem  mask(Virtual Unit Delay){}
      settings: AttributesFormatString=block has no effect
      mask Display: disp('1/z')
  n : Constant  Value=Samples  OutDataTypeStr=SamplesDataType
  y : Outport
  wires:
  Flip-Flop/1 -> VariantDebounce/2("tf "), Count/1(en)
  Virtual Unit Delay/1(y) -> OR/2
  u/1 -> VariantDebounce/1("u "), VariantControl/1("u ")
  OR/1 -> Flip-Flop/2
  VariantControl/1(set) -> Flip-Flop/1
  VariantControl/2(rs) -> OR/1
  n/1 -> Count/2(n)
  Count/1(rs) -> Virtual Unit Delay/1(u)
  VariantDebounce/1(" y") -> y/1

== system libbestfx/Signal Operations/Flip-Flop ==
  S : Inport
  R : Inport  Port=2
  !Q : Terminator
  Demux : Demux  Outputs=2
  Mux : Mux  Inputs=3
  Unit Delay : UnitDelay  InitialCondition=InitialCondition  SampleTime=-1
  VariantType : Subsystem  VariantControlMode=Label  Variant=on  VariantControl=Variant1  LabelModeActiveChoice=VariantTypeS-R
  Q : Outport
  wires:
  VariantType/1(" y") -> Demux/1
  Mux/1 -> VariantType/1("u ")
  R/1 -> Mux/2
  Unit Delay/1 -> Mux/3
  S/1 -> Mux/1
  Demux/1 -> Q/1, Unit Delay/1
  Demux/2 -> !Q/1

== system libbestfx/Signal Operations/Interactive Switch ==
  Constant1 : Constant  Value=ctrl  OutDataTypeStr=boolean  SampleTime=-1
  Constant3 : Constant  OutDataTypeStr=boolean
  Constant4 : Constant  Value=0  OutDataTypeStr=boolean
  Switch : Switch  Criteria=u2 ~= 0
  y : Outport
  wires:
  Switch/1 -> y/1
  Constant4/1 -> Switch/3
  Constant3/1 -> Switch/1
  Constant1/1 -> Switch/2

== system libbestfx/Signal Operations/Pulse Divider ==
  u : Inport
  Data Type Duplicate : DataTypeDuplicate
  Detect Increase : simulink/Logic and Bit Operations/Detect Increase  vinit=0.0  OutDataTypeStr=boolean
  Edge Counter : Subsystem
  Relational Operator : RelationalOperator  OutDataTypeStr=boolean  RndMeth=Simplest
  Toggle : Subsystem
  k : Constant  Value=Divisor  OutDataTypeStr=DivisorDataType
  y : Outport
  wires:
  Edge Counter/1(cntr) -> Relational Operator/1
  Toggle/1(y) -> y/1, Data Type Duplicate/2
  Relational Operator/1 -> Toggle/1(u)
  k/1 -> Edge Counter/2(k), Relational Operator/2
  u/1 -> Detect Increase/1, Data Type Duplicate/1
  Detect Increase/1 -> Edge Counter/1(edge)

== system libbestfx/Signal Operations/Pulse Selector ==
  u : Inport
  Detect Decrease : simulink/Logic and Bit Operations/Detect Decrease  vinit=0.0  OutDataTypeStr=boolean
  Detect Increase : simulink/Logic and Bit Operations/Detect Increase  vinit=0.0  OutDataTypeStr=boolean
  Edge Counter : Subsystem
  Relational Operator : RelationalOperator  Operator=>  OutDataTypeStr=boolean  RndMeth=Simplest
  Switch To Zero : $bdroot/Signal Operations/Switch To Zero
  n : Constant  Value=Subset  OutDataTypeStr=SubsetDataType
  nmax : Constant  Value=Maximum  OutDataTypeStr=MaximumDataType
  y : Outport
  wires:
  Relational Operator/1 -> Switch To Zero/2
  Detect Decrease/1 -> Edge Counter/2(edge_neg)
  n/1 -> Relational Operator/2
  nmax/1 -> Edge Counter/3(k)
  Switch To Zero/1 -> y/1
  Detect Increase/1 -> Edge Counter/1(edge_pos)
  Edge Counter/1(cntr) -> Relational Operator/1
  u/1 -> Detect Increase/1, Detect Decrease/1, Switch To Zero/1

== system libbestfx/Signal Operations/Switch To Zero ==
  u : Inport
  TF : Inport  Port=2
  Overwrite : $bdroot/Signal Attributes/Overwrite  val=0.0
  Switch : Switch  Criteria=u2 > Threshold
      settings: AttributesFormatString=%<Criteria> \n Threshold: %<Threshold>
  y : Outport  OutputWhenDisabled=reset  InitialOutput=[0]
  wires:
  Switch/1 -> y/1
  u/1 -> Overwrite/1, Switch/3
  TF/1 -> Switch/2
  Overwrite/1 -> Switch/1

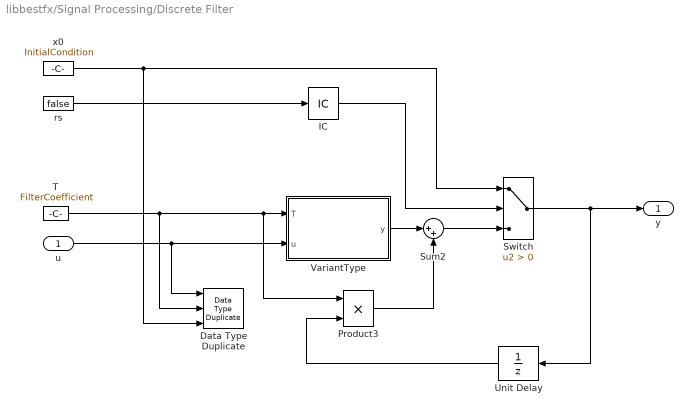
== system libbestfx/Signal Processing/Discrete Filter ==
  u : Inport
  Data Type Duplicate : DataTypeDuplicate  NumInputPorts=3
  IC : InitialCondition
  Product3 : Product
  Sum2 : Sum  Inputs=|++
  Switch : Switch  Criteria=u2 > Threshold
      settings: AttributesFormatString=%<Criteria> \n Threshold: %<Threshold>
  T : Constant  Value=FilterCoefficient  OutDataTypeStr=FilterCoefficientDataType
  Unit Delay : UnitDelay  SampleTime=-1
  VariantType : Subsystem  VariantControlMode=Label  Variant=on  VariantControl=Variant1  LabelModeActiveChoice=VariantTypeLowpass
  rs : Constant  Value=false
  x0 : Constant  Value=InitialCondition  OutDataTypeStr=InitialConditionDataType
  y : Outport
  wires:
  Sum2/1 -> Switch/3
  rs/1 -> IC/1
  IC/1 -> Switch/2
  x0/1 -> Data Type Duplicate/3, Switch/1
  T/1 -> Data Type Duplicate/2, Product3/1, VariantType/1("T ")
  Switch/1 -> y/1, Unit Delay/1
  u/1 -> Data Type Duplicate/1, VariantType/2("u ")
  Product3/1 -> Sum2/2
  Unit Delay/1 -> Product3/2
  VariantType/1(" y") -> Sum2/1

== system libbestfx/Signal Verification/Validate ==
  u : Inport
  VariantRange : Subsystem  VariantControlMode=Label  Variant=on  LabelModeActiveChoice=VariantRangeInside
  VariantType : Subsystem  VariantControlMode=Label  Variant=on  LabelModeActiveChoice=VariantTypePassThrough
  lwr : Constant  Value=LowerLimit  OutDataTypeStr=LowerLimitDataType
  upr : Constant  Value=UpperLimit  OutDataTypeStr=UpperLimitDataType
  valid : Outport
  wires:
  u/1 -> VariantType/2(u), VariantRange/1(u)
  lwr/1 -> VariantRange/2(lwr)
  upr/1 -> VariantRange/3(upr)
  VariantRange/1(state) -> VariantType/1(state)
  VariantType/1(valid) -> valid/1

== system libbestfx/Model Settings/Design Block/Empty ==

== system libbestfx/Signal Attributes/Data Pack/VariantSpecifier ==
  "u " : Inport
  PassThrough : Subsystem  VariantControl=VariantSpecifierPassThrough
  Signed : Subsystem  VariantControl=VariantSpecifierSigned
  Unsigned : Subsystem  VariantControl=VariantSpecifierUnsigned
  " y" : Outport

== system libbestfx/Signal Attributes/Data Unpack/VariantSpecifier ==
  "u " : Inport
  PassThrough : Subsystem  VariantControl=VariantSpecifierPassThrough
  Signed : Subsystem  VariantControl=VariantSpecifierSigned
  Unsigned : Subsystem  VariantControl=VariantSpecifierUnsigned
  " y" : Outport
